simulink model "StateLinearClosedLoop"  (Simulink 7.9)
settings: Solver=ode45  StartTime=0.0  StopTime=2.5  RelTol=1e-3
values from neighbouring files (symbols this model uses):
  A = [0 1 0; a21 a22 a23; a31 a32 a33]    [parameters.m]
  B = [0; b2; b3]    [parameters.m]
  C = [1 0 0; 0 1 0; 0 0 1]    [LQR.m]
  D = [0; 0; 0]    [LQR.m]
  K = lqr(A,B,Q,R)    [LQR.m]
settings Model: Creator=gdiazh  LastModifiedBy=root
settings OptimizationCC: InitFltsAndDblsToZero=on
settings DebuggingCC: FcnCallInpInsideContextMsg=Use local settings  StrictBusMsg=Warning
settings SFSimCC: SimParseCustomCode=off
settings GRTTargetCC: CombineOutputUpdateFcns=off  GRTInterface=on

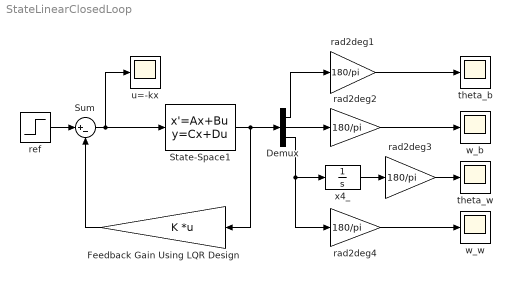
== system StateLinearClosedLoop ==
  Demux : Demux  Outputs=3
  Feedback Gain Using LQR Design : Gain  Gain=K  Multiplication=Matrix(K*u) (u vector)
  State-Space1 : StateSpace  A=A  B=B  C=C  D=D  X0=[10*pi/180; 10; 1 ]
  Sum : Sum  Inputs=|+-
  rad2deg{1..4} (4 alike) : Gain  Gain=180/pi  SaturateOnIntegerOverflow=on  OutDataTypeStr=Inherit: Same as input  ParamDataTypeStr=Inherit: Same as input
  ref : Step  Time=0  After=0  SampleTime=0
  theta_b : Scope
      settings: YMin=2e-07  YMax=2.5e-06  SaveName=position
  theta_w : Scope
      settings: SaveName=linealVel
  u=-kx : Scope
      settings: YMin=2e-07  YMax=2.5e-06  SaveName=position1
  w_b : Scope
      settings: TimeRange=0.35  YMin=88.25  YMax=91.75  SaveName=theta
  w_w : Scope
      settings: SaveName=angularVel
  x4_ : Integrator  UpperSaturationLimit=100  LowerSaturationLimit=-100
  wires:
  rad2deg4/1 -> w_w/1
  rad2deg1/1 -> theta_b/1
  rad2deg3/1 -> theta_w/1
  Demux/1 -> rad2deg1/1
  Demux/3 -> rad2deg4/1, x4_/1
  rad2deg2/1 -> w_b/1
  ref/1 -> Sum/1
  State-Space1/1 -> Demux/1, Feedback Gain Using LQR Design/1
  Demux/2 -> rad2deg2/1
  x4_/1 -> rad2deg3/1
  Sum/1 -> State-Space1/1, u=-kx/1
  Feedback Gain Using LQR Design/1 -> Sum/2
